simulink model "ModeloCorrea_Cinematico"  (R2023b)
settings: Solver=ode23  StartTime=0.0  StopTime=30  RelTol=1e-3
PreLoadFcn:
  | cargar_datos
model workspace: external: MATLAB File Data\Ensamblaje_Correa_v2_DataFile.m (data not in the file)
undefined symbols (not defined in the file): D, DiscIntNeverNeededParam, Floor, L, R, smiData, X, Y, Z
libraries: sm_lib x464, nesl_utility x23, simulink x8, fl_lib x8, SignalEditorBlockLib x1
(part 2 of 10)

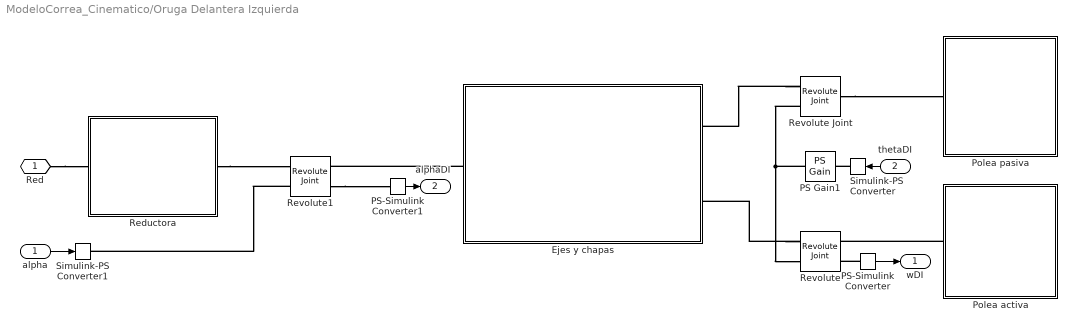
== system ModeloCorrea_Cinematico/Oruga Delantera Izquierda ==
  alpha : Inport
  thetaDI : Inport  Port=2
  Ejes y chapas : Subsystem
      mask Display: image('Ejes y chapas.png');
  PS Gain1 : fl_lib/Physical Signals/Functions/PS Gain  gain=-1
  PS-Simulink Converter : nesl_utility/PS-Simulink Converter  PhysicalDomain=network_engine_domain  SubClassName=ps_output  LeftPortType=input  RightPortType=output  PseudoPeriodic=off  Frequencies=[]  VectorFormat=inherit  Unit=rad/s  AffineConversion=off
  PS-Simulink Converter1 : nesl_utility/PS-Simulink Converter  PhysicalDomain=network_engine_domain  SubClassName=ps_output  LeftPortType=input  RightPortType=output  PseudoPeriodic=off  Frequencies=[]  VectorFormat=inherit  Unit=rad  AffineConversion=off
  Polea activa : Subsystem
      mask Display: image('Polea activa.png');
  Polea pasiva : Subsystem
      mask Display: image('Polea pasiva.png');
  Reductora : Subsystem
      mask Display: image('Reductora.png');
  Revolute : sm_lib/Joints/Revolute Joint  JointMode=Normal  SenseConstraintForce=off  SenseConstraintForceX=off  SenseConstraintForceY=off  SenseConstraintForceZ=off  SenseConstraintTorque=off  SenseConstraintTorqueX=off  SenseConstraintTorqueY=off  SenseConstraintTorqueZ=off  SenseTotalForce=off  SenseTotalForceX=off  SenseTotalForceY=off  SenseTotalForceZ=off  SenseTotalTorque=off  SenseTotalTorqueX=off  SenseTotalTorqueY=off  SenseTotalTorqueZ=off  CompositeWrenchDir=FollowerOnBase  CompositeWrenchFrame=BaseFrame  EquilibriumPosition=0  EquilibriumPositionUnits=deg  SpringStiffness=0  SpringStiffnessUnits=N*m/deg  DampingCoefficient=5e-4  DampingCoefficientUnits=N*m/(deg/s)  TorqueActuationMode=ComputedTorque  MotionActuationMode=InputMotion  SensePosition=off  SenseVelocity=on  SenseAcceleration=off  SenseTorqueForce=off  SenseLowerLimitTorqueForce=off  SenseUpperLimitTorqueForce=off  LowerLimitSpecify=off  LowerLimitBound=-90  LowerLimitBoundUnits=deg  LowerLimitStiffness=1e4  LowerLimitStiffnessUnits=N*m/deg  LowerLimitDamping=10  LowerLimitDampingUnits=N*m/(deg/s)  LowerLimitTransitionRegionWidth=0.1  LowerLimitTransitionRegionWidthUnits=deg  UpperLimitSpecify=off  UpperLimitBound=90  UpperLimitBoundUnits=deg  UpperLimitStiffness=1e4  UpperLimitStiffnessUnits=N*m/deg  UpperLimitDamping=10  UpperLimitDampingUnits=N*m/(deg/s)  UpperLimitTransitionRegionWidth=0.1  UpperLimitTransitionRegionWidthUnits=deg  PositionTargetSpecify=on  PositionTargetPriority=Low  PositionTargetValue=smiData.RevoluteJoint(1).Rz.Pos  PositionTargetValueUnits=deg  VelocityTargetSpecify=off  VelocityTargetPriority=High  VelocityTargetValue=0  VelocityTargetValueUnits=deg/s
  Revolute Joint : sm_lib/Joints/Revolute Joint  JointMode=Normal  SenseConstraintForce=off  SenseConstraintForceX=off  SenseConstraintForceY=off  SenseConstraintForceZ=off  SenseConstraintTorque=off  SenseConstraintTorqueX=off  SenseConstraintTorqueY=off  SenseConstraintTorqueZ=off  SenseTotalForce=off  SenseTotalForceX=off  SenseTotalForceY=off  SenseTotalForceZ=off  SenseTotalTorque=off  SenseTotalTorqueX=off  SenseTotalTorqueY=off  SenseTotalTorqueZ=off  CompositeWrenchDir=FollowerOnBase  CompositeWrenchFrame=BaseFrame  EquilibriumPosition=0  EquilibriumPositionUnits=deg  SpringStiffness=0  SpringStiffnessUnits=N*m/deg  DampingCoefficient=5e-4  DampingCoefficientUnits=N*m/(deg/s)  TorqueActuationMode=ComputedTorque  MotionActuationMode=InputMotion  SensePosition=off  SenseVelocity=off  SenseAcceleration=off  SenseTorqueForce=off  SenseLowerLimitTorqueForce=off  SenseUpperLimitTorqueForce=off  LowerLimitSpecify=off  LowerLimitBound=-90  LowerLimitBoundUnits=deg  LowerLimitStiffness=1e4  LowerLimitStiffnessUnits=N*m/deg  LowerLimitDamping=10  LowerLimitDampingUnits=N*m/(deg/s)  LowerLimitTransitionRegionWidth=0.1  LowerLimitTransitionRegionWidthUnits=deg  UpperLimitSpecify=off  UpperLimitBound=90  UpperLimitBoundUnits=deg  UpperLimitStiffness=1e4  UpperLimitStiffnessUnits=N*m/deg  UpperLimitDamping=10  UpperLimitDampingUnits=N*m/(deg/s)  UpperLimitTransitionRegionWidth=0.1  UpperLimitTransitionRegionWidthUnits=deg  PositionTargetSpecify=off  PositionTargetPriority=High  PositionTargetValue=0  PositionTargetValueUnits=deg  VelocityTargetSpecify=off  VelocityTargetPriority=High  VelocityTargetValue=0  VelocityTargetValueUnits=deg/s
  Revolute1 : sm_lib/Joints/Revolute Joint  JointMode=Normal  SenseConstraintForce=off  SenseConstraintForceX=off  SenseConstraintForceY=off  SenseConstraintForceZ=off  SenseConstraintTorque=off  SenseConstraintTorqueX=off  SenseConstraintTorqueY=off  SenseConstraintTorqueZ=off  SenseTotalForce=off  SenseTotalForceX=off  SenseTotalForceY=off  SenseTotalForceZ=off  SenseTotalTorque=off  SenseTotalTorqueX=off  SenseTotalTorqueY=off  SenseTotalTorqueZ=off  CompositeWrenchDir=FollowerOnBase  CompositeWrenchFrame=BaseFrame  EquilibriumPosition=0  EquilibriumPositionUnits=deg  SpringStiffness=0  SpringStiffnessUnits=N*m/deg  DampingCoefficient=5e-4  DampingCoefficientUnits=N*m/(deg/s)  TorqueActuationMode=ComputedTorque  MotionActuationMode=InputMotion  SensePosition=on  SenseVelocity=off  SenseAcceleration=off  SenseTorqueForce=off  SenseLowerLimitTorqueForce=off  SenseUpperLimitTorqueForce=off  LowerLimitSpecify=on  LowerLimitBound=0  LowerLimitBoundUnits=deg  LowerLimitStiffness=1e4  LowerLimitStiffnessUnits=N*m/deg  LowerLimitDamping=10  LowerLimitDampingUnits=N*m/(deg/s)  LowerLimitTransitionRegionWidth=0.1  LowerLimitTransitionRegionWidthUnits=deg  UpperLimitSpecify=on  UpperLimitBound=90  UpperLimitBoundUnits=deg  UpperLimitStiffness=1e4  UpperLimitStiffnessUnits=N*m/deg  UpperLimitDamping=10  UpperLimitDampingUnits=N*m/(deg/s)  UpperLimitTransitionRegionWidth=0.1  UpperLimitTransitionRegionWidthUnits=deg  PositionTargetSpecify=on  PositionTargetPriority=Low  PositionTargetValue=smiData.RevoluteJoint(2).Rz.Pos  PositionTargetValueUnits=deg  VelocityTargetSpecify=off  VelocityTargetPriority=High  VelocityTargetValue=0  VelocityTargetValueUnits=deg/s
  Simulink-PS Converter : nesl_utility/Simulink-PS Converter  PhysicalDomain=network_engine_domain  SubClassName=ps_input  LeftPortType=input  RightPortType=output  PseudoPeriodic=off  Frequencies=[]  NoiseDistribution=none  NoiseParameters=[]  Unit=1  AffineConversion=off  FilteringAndDerivatives=filter  SimscapeFilterOrder=2  InputFilterTimeConstant=0.001  UdotUserProvided=0
  Simulink-PS Converter1 : nesl_utility/Simulink-PS Converter  PhysicalDomain=network_engine_domain  SubClassName=ps_input  LeftPortType=input  RightPortType=output  PseudoPeriodic=off  Frequencies=[]  NoiseDistribution=none  NoiseParameters=[]  Unit=1  AffineConversion=off  FilteringAndDerivatives=filter  SimscapeFilterOrder=2  InputFilterTimeConstant=0.001  UdotUserProvided=0
  Red : PMIOPort  Side=Left
  wDI : Outport
  alphaDI : Outport  Port=2
  wires:
  thetaDI/1 -> Simulink-PS Converter/1
  PS-Simulink Converter/1 -> wDI/1
  alpha/1 -> Simulink-PS Converter1/1
  PS-Simulink Converter1/1 -> alphaDI/1
  connections:
  Red/RConn1 -- Reductora/LConn1
  Ejes y chapas/LConn1 -- Revolute1/RConn1
  Reductora/RConn1 -- Revolute1/LConn1
  Polea activa/LConn1 -- Revolute/RConn1
  Revolute/LConn1 -- Ejes y chapas/RConn2
  Revolute Joint/RConn1 -- Polea pasiva/LConn1
  Revolute Joint/LConn1 -- Ejes y chapas/RConn1
  PS Gain1/RConn1 -- Revolute/LConn2 -- Revolute Joint/LConn2
  PS-Simulink Converter/LConn1 -- Revolute/RConn2
  Revolute1/LConn2 -- Simulink-PS Converter1/RConn1
  Revolute1/RConn2 -- PS-Simulink Converter1/LConn1
  Simulink-PS Converter/RConn1 -- PS Gain1/LConn1

== system ModeloCorrea_Cinematico/Oruga Trasera Derecha ==
  alpha : Inport
  thetaTD : Inport  Port=2
  Ejes y chapas : Subsystem
      mask Display: image('Ejes y chapas.png');
  PS Gain1 : fl_lib/Physical Signals/Functions/PS Gain  gain=-1
  PS-Simulink Converter : nesl_utility/PS-Simulink Converter  PhysicalDomain=network_engine_domain  SubClassName=ps_output  LeftPortType=input  RightPortType=output  PseudoPeriodic=off  Frequencies=[]  VectorFormat=inherit  Unit=rad/s  AffineConversion=off
  PS-Simulink Converter1 : nesl_utility/PS-Simulink Converter  PhysicalDomain=network_engine_domain  SubClassName=ps_output  LeftPortType=input  RightPortType=output  PseudoPeriodic=off  Frequencies=[]  VectorFormat=inherit  Unit=rad  AffineConversion=off
  Polea activa : Subsystem
      mask Display: image('Polea activa.png');
  Polea pasiva : Subsystem
      mask Display: image('Polea pasiva.png');
  Reductora : Subsystem
      mask Display: image('Reductora.png');
  Revolute : sm_lib/Joints/Revolute Joint  JointMode=Normal  SenseConstraintForce=off  SenseConstraintForceX=off  SenseConstraintForceY=off  SenseConstraintForceZ=off  SenseConstraintTorque=off  SenseConstraintTorqueX=off  SenseConstraintTorqueY=off  SenseConstraintTorqueZ=off  SenseTotalForce=off  SenseTotalForceX=off  SenseTotalForceY=off  SenseTotalForceZ=off  SenseTotalTorque=off  SenseTotalTorqueX=off  SenseTotalTorqueY=off  SenseTotalTorqueZ=off  CompositeWrenchDir=FollowerOnBase  CompositeWrenchFrame=BaseFrame  EquilibriumPosition=0  EquilibriumPositionUnits=deg  SpringStiffness=0  SpringStiffnessUnits=N*m/deg  DampingCoefficient=5e-4  DampingCoefficientUnits=N*m/(deg/s)  TorqueActuationMode=ComputedTorque  MotionActuationMode=InputMotion  SensePosition=off  SenseVelocity=on  SenseAcceleration=off  SenseTorqueForce=off  SenseLowerLimitTorqueForce=off  SenseUpperLimitTorqueForce=off  LowerLimitSpecify=off  LowerLimitBound=-90  LowerLimitBoundUnits=deg  LowerLimitStiffness=1e4  LowerLimitStiffnessUnits=N*m/deg  LowerLimitDamping=10  LowerLimitDampingUnits=N*m/(deg/s)  LowerLimitTransitionRegionWidth=0.1  LowerLimitTransitionRegionWidthUnits=deg  UpperLimitSpecify=off  UpperLimitBound=90  UpperLimitBoundUnits=deg  UpperLimitStiffness=1e4  UpperLimitStiffnessUnits=N*m/deg  UpperLimitDamping=10  UpperLimitDampingUnits=N*m/(deg/s)  UpperLimitTransitionRegionWidth=0.1  UpperLimitTransitionRegionWidthUnits=deg  PositionTargetSpecify=on  PositionTargetPriority=Low  PositionTargetValue=smiData.RevoluteJoint(1).Rz.Pos  PositionTargetValueUnits=deg  VelocityTargetSpecify=off  VelocityTargetPriority=High  VelocityTargetValue=0  VelocityTargetValueUnits=deg/s
  Revolute Joint : sm_lib/Joints/Revolute Joint  JointMode=Normal  SenseConstraintForce=off  SenseConstraintForceX=off  SenseConstraintForceY=off  SenseConstraintForceZ=off  SenseConstraintTorque=off  SenseConstraintTorqueX=off  SenseConstraintTorqueY=off  SenseConstraintTorqueZ=off  SenseTotalForce=off  SenseTotalForceX=off  SenseTotalForceY=off  SenseTotalForceZ=off  SenseTotalTorque=off  SenseTotalTorqueX=off  SenseTotalTorqueY=off  SenseTotalTorqueZ=off  CompositeWrenchDir=FollowerOnBase  CompositeWrenchFrame=BaseFrame  EquilibriumPosition=0  EquilibriumPositionUnits=deg  SpringStiffness=0  SpringStiffnessUnits=N*m/deg  DampingCoefficient=5e-4  DampingCoefficientUnits=N*m/(deg/s)  TorqueActuationMode=ComputedTorque  MotionActuationMode=InputMotion  SensePosition=off  SenseVelocity=off  SenseAcceleration=off  SenseTorqueForce=off  SenseLowerLimitTorqueForce=off  SenseUpperLimitTorqueForce=off  LowerLimitSpecify=off  LowerLimitBound=-90  LowerLimitBoundUnits=deg  LowerLimitStiffness=1e4  LowerLimitStiffnessUnits=N*m/deg  LowerLimitDamping=10  LowerLimitDampingUnits=N*m/(deg/s)  LowerLimitTransitionRegionWidth=0.1  LowerLimitTransitionRegionWidthUnits=deg  UpperLimitSpecify=off  UpperLimitBound=90  UpperLimitBoundUnits=deg  UpperLimitStiffness=1e4  UpperLimitStiffnessUnits=N*m/deg  UpperLimitDamping=10  UpperLimitDampingUnits=N*m/(deg/s)  UpperLimitTransitionRegionWidth=0.1  UpperLimitTransitionRegionWidthUnits=deg  PositionTargetSpecify=off  PositionTargetPriority=High  PositionTargetValue=0  PositionTargetValueUnits=deg  VelocityTargetSpecify=off  VelocityTargetPriority=High  VelocityTargetValue=0  VelocityTargetValueUnits=deg/s
  Revolute1 : sm_lib/Joints/Revolute Joint  JointMode=Normal  SenseConstraintForce=off  SenseConstraintForceX=off  SenseConstraintForceY=off  SenseConstraintForceZ=off  SenseConstraintTorque=off  SenseConstraintTorqueX=off  SenseConstraintTorqueY=off  SenseConstraintTorqueZ=off  SenseTotalForce=off  SenseTotalForceX=off  SenseTotalForceY=off  SenseTotalForceZ=off  SenseTotalTorque=off  SenseTotalTorqueX=off  SenseTotalTorqueY=off  SenseTotalTorqueZ=off  CompositeWrenchDir=FollowerOnBase  CompositeWrenchFrame=BaseFrame  EquilibriumPosition=0  EquilibriumPositionUnits=deg  SpringStiffness=0  SpringStiffnessUnits=N*m/deg  DampingCoefficient=5e-4  DampingCoefficientUnits=N*m/(deg/s)  TorqueActuationMode=ComputedTorque  MotionActuationMode=InputMotion  SensePosition=on  SenseVelocity=off  SenseAcceleration=off  SenseTorqueForce=off  SenseLowerLimitTorqueForce=off  SenseUpperLimitTorqueForce=off  LowerLimitSpecify=on  LowerLimitBound=0  LowerLimitBoundUnits=deg  LowerLimitStiffness=1e4  LowerLimitStiffnessUnits=N*m/deg  LowerLimitDamping=10  LowerLimitDampingUnits=N*m/(deg/s)  LowerLimitTransitionRegionWidth=0.1  LowerLimitTransitionRegionWidthUnits=deg  UpperLimitSpecify=on  UpperLimitBound=90  UpperLimitBoundUnits=deg  UpperLimitStiffness=1e4  UpperLimitStiffnessUnits=N*m/deg  UpperLimitDamping=10  UpperLimitDampingUnits=N*m/(deg/s)  UpperLimitTransitionRegionWidth=0.1  UpperLimitTransitionRegionWidthUnits=deg  PositionTargetSpecify=on  PositionTargetPriority=Low  PositionTargetValue=smiData.RevoluteJoint(2).Rz.Pos  PositionTargetValueUnits=deg  VelocityTargetSpecify=off  VelocityTargetPriority=High  VelocityTargetValue=0  VelocityTargetValueUnits=deg/s
  Simulink-PS Converter : nesl_utility/Simulink-PS Converter  PhysicalDomain=network_engine_domain  SubClassName=ps_input  LeftPortType=input  RightPortType=output  PseudoPeriodic=off  Frequencies=[]  NoiseDistribution=none  NoiseParameters=[]  Unit=1  AffineConversion=off  FilteringAndDerivatives=filter  SimscapeFilterOrder=2  InputFilterTimeConstant=0.001  UdotUserProvided=0
  Simulink-PS Converter1 : nesl_utility/Simulink-PS Converter  PhysicalDomain=network_engine_domain  SubClassName=ps_input  LeftPortType=input  RightPortType=output  PseudoPeriodic=off  Frequencies=[]  NoiseDistribution=none  NoiseParameters=[]  Unit=1  AffineConversion=off  FilteringAndDerivatives=filter  SimscapeFilterOrder=2  InputFilterTimeConstant=0.001  UdotUserProvided=0
  Red : PMIOPort  Side=Left
  wTD : Outport
  alphaTD : Outport  Port=2
  wires:
  thetaTD/1 -> Simulink-PS Converter/1
  PS-Simulink Converter/1 -> wTD/1
  alpha/1 -> Simulink-PS Converter1/1
  PS-Simulink Converter1/1 -> alphaTD/1
  connections:
  Red/RConn1 -- Reductora/LConn1
  Ejes y chapas/LConn1 -- Revolute1/RConn1
  Reductora/RConn1 -- Revolute1/LConn1
  Polea activa/LConn1 -- Revolute/RConn1
  Revolute/LConn1 -- Ejes y chapas/RConn2
  Revolute Joint/RConn1 -- Polea pasiva/LConn1
  Revolute Joint/LConn1 -- Ejes y chapas/RConn1
  Revolute Joint/LConn2 -- Revolute/LConn2 -- PS Gain1/RConn1
  PS-Simulink Converter/LConn1 -- Revolute/RConn2
  Simulink-PS Converter1/RConn1 -- Revolute1/LConn2
  Revolute1/RConn2 -- PS-Simulink Converter1/LConn1
  Simulink-PS Converter/RConn1 -- PS Gain1/LConn1

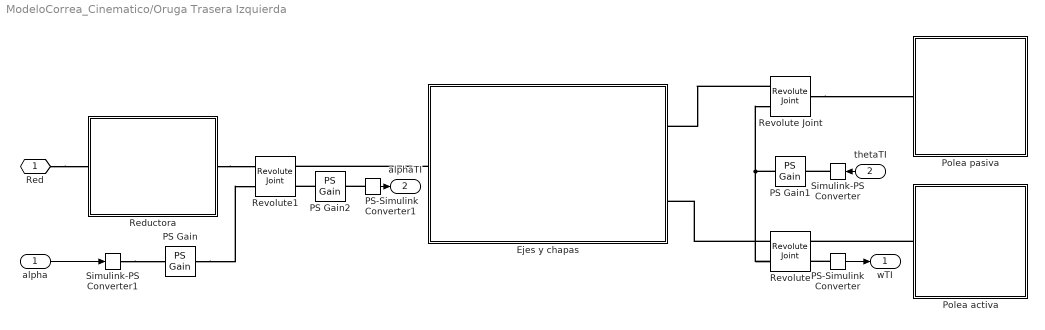
== system ModeloCorrea_Cinematico/Oruga Trasera Izquierda ==
  alpha : Inport
  thetaTI : Inport  Port=2
  Ejes y chapas : Subsystem
      mask Display: image('Ejes y chapas.png');
  PS Gain : fl_lib/Physical Signals/Functions/PS Gain  gain=-1
  PS Gain1 : fl_lib/Physical Signals/Functions/PS Gain  gain=-1
  PS Gain2 : fl_lib/Physical Signals/Functions/PS Gain  gain=-1
  PS-Simulink Converter : nesl_utility/PS-Simulink Converter  PhysicalDomain=network_engine_domain  SubClassName=ps_output  LeftPortType=input  RightPortType=output  PseudoPeriodic=off  Frequencies=[]  VectorFormat=inherit  Unit=rad/s  AffineConversion=off
  PS-Simulink Converter1 : nesl_utility/PS-Simulink Converter  PhysicalDomain=network_engine_domain  SubClassName=ps_output  LeftPortType=input  RightPortType=output  PseudoPeriodic=off  Frequencies=[]  VectorFormat=inherit  Unit=rad  AffineConversion=off
  Polea activa : Subsystem
      mask Display: image('Polea activa.png');
  Polea pasiva : Subsystem
      mask Display: image('Polea pasiva.png');
  Reductora : Subsystem
      mask Display: image('Reductora.png');
  Revolute : sm_lib/Joints/Revolute Joint  JointMode=Normal  SenseConstraintForce=off  SenseConstraintForceX=off  SenseConstraintForceY=off  SenseConstraintForceZ=off  SenseConstraintTorque=off  SenseConstraintTorqueX=off  SenseConstraintTorqueY=off  SenseConstraintTorqueZ=off  SenseTotalForce=off  SenseTotalForceX=off  SenseTotalForceY=off  SenseTotalForceZ=off  SenseTotalTorque=off  SenseTotalTorqueX=off  SenseTotalTorqueY=off  SenseTotalTorqueZ=off  CompositeWrenchDir=FollowerOnBase  CompositeWrenchFrame=BaseFrame  EquilibriumPosition=0  EquilibriumPositionUnits=deg  SpringStiffness=0  SpringStiffnessUnits=N*m/deg  DampingCoefficient=5e-4  DampingCoefficientUnits=N*m/(deg/s)  TorqueActuationMode=ComputedTorque  MotionActuationMode=InputMotion  SensePosition=off  SenseVelocity=on  SenseAcceleration=off  SenseTorqueForce=off  SenseLowerLimitTorqueForce=off  SenseUpperLimitTorqueForce=off  LowerLimitSpecify=off  LowerLimitBound=-90  LowerLimitBoundUnits=deg  LowerLimitStiffness=1e4  LowerLimitStiffnessUnits=N*m/deg  LowerLimitDamping=10  LowerLimitDampingUnits=N*m/(deg/s)  LowerLimitTransitionRegionWidth=0.1  LowerLimitTransitionRegionWidthUnits=deg  UpperLimitSpecify=off  UpperLimitBound=90  UpperLimitBoundUnits=deg  UpperLimitStiffness=1e4  UpperLimitStiffnessUnits=N*m/deg  UpperLimitDamping=10  UpperLimitDampingUnits=N*m/(deg/s)  UpperLimitTransitionRegionWidth=0.1  UpperLimitTransitionRegionWidthUnits=deg  PositionTargetSpecify=on  PositionTargetPriority=Low  PositionTargetValue=smiData.RevoluteJoint(1).Rz.Pos  PositionTargetValueUnits=deg  VelocityTargetSpecify=off  VelocityTargetPriority=High  VelocityTargetValue=0  VelocityTargetValueUnits=deg/s
  Revolute Joint : sm_lib/Joints/Revolute Joint  JointMode=Normal  SenseConstraintForce=off  SenseConstraintForceX=off  SenseConstraintForceY=off  SenseConstraintForceZ=off  SenseConstraintTorque=off  SenseConstraintTorqueX=off  SenseConstraintTorqueY=off  SenseConstraintTorqueZ=off  SenseTotalForce=off  SenseTotalForceX=off  SenseTotalForceY=off  SenseTotalForceZ=off  SenseTotalTorque=off  SenseTotalTorqueX=off  SenseTotalTorqueY=off  SenseTotalTorqueZ=off  CompositeWrenchDir=FollowerOnBase  CompositeWrenchFrame=BaseFrame  EquilibriumPosition=0  EquilibriumPositionUnits=deg  SpringStiffness=0  SpringStiffnessUnits=N*m/deg  DampingCoefficient=5e-4  DampingCoefficientUnits=N*m/(deg/s)  TorqueActuationMode=ComputedTorque  MotionActuationMode=InputMotion  SensePosition=off  SenseVelocity=off  SenseAcceleration=off  SenseTorqueForce=off  SenseLowerLimitTorqueForce=off  SenseUpperLimitTorqueForce=off  LowerLimitSpecify=off  LowerLimitBound=-90  LowerLimitBoundUnits=deg  LowerLimitStiffness=1e4  LowerLimitStiffnessUnits=N*m/deg  LowerLimitDamping=10  LowerLimitDampingUnits=N*m/(deg/s)  LowerLimitTransitionRegionWidth=0.1  LowerLimitTransitionRegionWidthUnits=deg  UpperLimitSpecify=off  UpperLimitBound=90  UpperLimitBoundUnits=deg  UpperLimitStiffness=1e4  UpperLimitStiffnessUnits=N*m/deg  UpperLimitDamping=10  UpperLimitDampingUnits=N*m/(deg/s)  UpperLimitTransitionRegionWidth=0.1  UpperLimitTransitionRegionWidthUnits=deg  PositionTargetSpecify=off  PositionTargetPriority=High  PositionTargetValue=0  PositionTargetValueUnits=deg  VelocityTargetSpecify=off  VelocityTargetPriority=High  VelocityTargetValue=0  VelocityTargetValueUnits=deg/s
  Revolute1 : sm_lib/Joints/Revolute Joint  JointMode=Normal  SenseConstraintForce=off  SenseConstraintForceX=off  SenseConstraintForceY=off  SenseConstraintForceZ=off  SenseConstraintTorque=off  SenseConstraintTorqueX=off  SenseConstraintTorqueY=off  SenseConstraintTorqueZ=off  SenseTotalForce=off  SenseTotalForceX=off  SenseTotalForceY=off  SenseTotalForceZ=off  SenseTotalTorque=off  SenseTotalTorqueX=off  SenseTotalTorqueY=off  SenseTotalTorqueZ=off  CompositeWrenchDir=FollowerOnBase  CompositeWrenchFrame=BaseFrame  EquilibriumPosition=0  EquilibriumPositionUnits=deg  SpringStiffness=0  SpringStiffnessUnits=N*m/deg  DampingCoefficient=5e-4  DampingCoefficientUnits=N*m/(deg/s)  TorqueActuationMode=ComputedTorque  MotionActuationMode=InputMotion  SensePosition=on  SenseVelocity=off  SenseAcceleration=off  SenseTorqueForce=off  SenseLowerLimitTorqueForce=off  SenseUpperLimitTorqueForce=off  LowerLimitSpecify=on  LowerLimitBound=0  LowerLimitBoundUnits=deg  LowerLimitStiffness=1e4  LowerLimitStiffnessUnits=N*m/deg  LowerLimitDamping=10  LowerLimitDampingUnits=N*m/(deg/s)  LowerLimitTransitionRegionWidth=0.1  LowerLimitTransitionRegionWidthUnits=deg  UpperLimitSpecify=on  UpperLimitBound=90  UpperLimitBoundUnits=deg  UpperLimitStiffness=1e4  UpperLimitStiffnessUnits=N*m/deg  UpperLimitDamping=10  UpperLimitDampingUnits=N*m/(deg/s)  UpperLimitTransitionRegionWidth=0.1  UpperLimitTransitionRegionWidthUnits=deg  PositionTargetSpecify=on  PositionTargetPriority=Low  PositionTargetValue=smiData.RevoluteJoint(2).Rz.Pos  PositionTargetValueUnits=deg  VelocityTargetSpecify=off  VelocityTargetPriority=High  VelocityTargetValue=0  VelocityTargetValueUnits=deg/s
  Simulink-PS Converter : nesl_utility/Simulink-PS Converter  PhysicalDomain=network_engine_domain  SubClassName=ps_input  LeftPortType=input  RightPortType=output  PseudoPeriodic=off  Frequencies=[]  NoiseDistribution=none  NoiseParameters=[]  Unit=1  AffineConversion=off  FilteringAndDerivatives=filter  SimscapeFilterOrder=2  InputFilterTimeConstant=0.001  UdotUserProvided=0
  Simulink-PS Converter1 : nesl_utility/Simulink-PS Converter  PhysicalDomain=network_engine_domain  SubClassName=ps_input  LeftPortType=input  RightPortType=output  PseudoPeriodic=off  Frequencies=[]  NoiseDistribution=none  NoiseParameters=[]  Unit=1  AffineConversion=off  FilteringAndDerivatives=filter  SimscapeFilterOrder=2  InputFilterTimeConstant=0.001  UdotUserProvided=0
  Red : PMIOPort  Side=Left
  wTI : Outport
  alphaTI : Outport  Port=2
  wires:
  thetaTI/1 -> Simulink-PS Converter/1
  PS-Simulink Converter/1 -> wTI/1
  alpha/1 -> Simulink-PS Converter1/1
  PS-Simulink Converter1/1 -> alphaTI/1
  connections:
  Red/RConn1 -- Reductora/LConn1
  Ejes y chapas/LConn1 -- Revolute1/RConn1
  Reductora/RConn1 -- Revolute1/LConn1
  Polea activa/LConn1 -- Revolute/RConn1
  Revolute/LConn1 -- Ejes y chapas/RConn2
  Revolute Joint/RConn1 -- Polea pasiva/LConn1
  PS Gain/RConn1 -- Revolute1/LConn2
  Revolute Joint/LConn1 -- Ejes y chapas/RConn1
  Revolute/LConn2 -- Revolute Joint/LConn2 -- PS Gain1/RConn1
  PS-Simulink Converter/LConn1 -- Revolute/RConn2
  PS-Simulink Converter1/LConn1 -- PS Gain2/RConn1
  Simulink-PS Converter1/RConn1 -- PS Gain/LConn1
  Simulink-PS Converter/RConn1 -- PS Gain1/LConn1
  PS Gain2/LConn1 -- Revolute1/RConn2

== system ModeloCorrea_Cinematico/Suelo ==
  Brick Solid : sm_lib/Body Elements/Brick Solid  GraphicAmbientColor=[0.15 0.15 0.15 1.0]  BasedOnType=Density  BrickDimensions=[Floor.l , Floor.w , Floor.h]  BrickDimensionsUnits=m  CenterOfMass=[0 0 0]  CenterOfMassUnits=m  GraphicDiffuseColor=[0.8 0.8 0.8]  Density=1000  DensityUnits=kg/m^3  DoExposeReferenceFrame=on  GraphicEmissiveColor=[0.0 0.0 0.0 1.0]  ExportEntireGeometry=off  SerializedFrames=<Frames/>  MarkerShape=Sphere  MarkerSize=10  GraphicType=FromGeometry  InertiaType=CalculateFromGeometry  Mass=1  MassUnits=kg  MomentsOfInertia=[1 1 1]  MomentsOfInertiaUnits=kg*m^2  GraphicOpacity=1.0  ProductsOfInertia=[0 0 0]  ProductsOfInertiaUnits=kg*m^2  GraphicShininess=75  GraphicSpecularColor=[0.5 0.5 0.5 1.0]  GraphicVisPropType=SimpleVisualProperties
  Extruded Solid : sm_lib/Body Elements/Extruded Solid  GraphicAmbientColor=[0.15 0.15 0.15 1.0]  BasedOnType=Density  CenterOfMass=[0 0 0]  CenterOfMassUnits=m  GraphicDiffuseColor=[0.4 0.4 0.4]  ExportConvexHullGeometry=off  ExtrusionCrossSection=Grid.extr_data  ExtrusionCrossSectionUnits=m  Density=1000  DensityUnits=kg/m^3  DoExposeReferenceFrame=on  GraphicEmissiveColor=[0.0 0.0 0.0 1.0]  ExportEntireGeometry=off  ExtrusionLength=Floor.h*1.005  ExtrusionLengthUnits=m  ExtrusionType=General  SerializedFrames=<Frames/>  MarkerShape=Sphere  MarkerSize=10  GraphicType=FromGeometry  InertiaType=CalculateFromGeometry  Mass=1  MassUnits=kg  MomentsOfInertia=[1 1 1]  MomentsOfInertiaUnits=kg*m^2  PolygonNumSides=3  GraphicOpacity=1.0  PolygonOuterRadius=1  PolygonOuterRadiusUnits=m  ProductsOfInertia=[0 0 0]  ProductsOfInertiaUnits=kg*m^2  GraphicShininess=75  GraphicSpecularColor=[0.5 0.5 0.5 1.0]  GraphicVisPropType=SimpleVisualProperties
  Extruded Solid1 : sm_lib/Body Elements/Extruded Solid  GraphicAmbientColor=[0.15 0.15 0.15 1.0]  BasedOnType=Density  CenterOfMass=[0 0 0]  CenterOfMassUnits=m  GraphicDiffuseColor=[0.4 0.4 0.4]  ExportConvexHullGeometry=off  ExtrusionCrossSection=Grid.extr_data  ExtrusionCrossSectionUnits=m  Density=1000  DensityUnits=kg/m^3  DoExposeReferenceFrame=on  GraphicEmissiveColor=[0.0 0.0 0.0 1.0]  ExportEntireGeometry=off  ExtrusionLength=Floor.h*1.005  ExtrusionLengthUnits=m  ExtrusionType=General  SerializedFrames=<Frames/>  MarkerShape=Sphere  MarkerSize=10  GraphicType=FromGeometry  InertiaType=CalculateFromGeometry  Mass=1  MassUnits=kg  MomentsOfInertia=[1 1 1]  MomentsOfInertiaUnits=kg*m^2  PolygonNumSides=3  GraphicOpacity=1.0  PolygonOuterRadius=1  PolygonOuterRadiusUnits=m  ProductsOfInertia=[0 0 0]  ProductsOfInertiaUnits=kg*m^2  GraphicShininess=75  GraphicSpecularColor=[0.5 0.5 0.5 1.0]  GraphicVisPropType=SimpleVisualProperties
  Rigid Transform1 : sm_lib/Frames and Transforms/Rigid Transform  TranslationMethod=None  TranslationStandardOffset=0  TranslationStandardOffsetUnits=m  TranslationStandardAxis=+Z  TranslationCartesianOffset=[0 0 0]  TranslationCartesianOffsetUnits=m  TranslationROffset=0  TranslationROffsetUnits=m  TranslationZOffset=0  TranslationZOffsetUnits=m  TranslationThetaOffset=0  TranslationThetaOffsetUnits=deg  RotationMethod=StandardAxis  RotationAngleUnits=deg  RotationStandardAxis=+Z  RotationAngle=90  RotationArbitraryAxis=[0 0 1]  FollAlignAxisA=+X  BaseAlignAxisA=+Y  FollAlignAxisB=+Y  BaseAlignAxisB=+Z  RotationSequenceAxes=FollowerAxes  RotationSequence=XYX  RotationSequenceAngles=[90 90 0]  RotationSequenceAnglesUnits=deg  RotationMatrix=[1 0 0; 0 1 0; 0 0 1]  Quaternion=[1 0 0 0]
  Input : PMIOPort  Side=Left
  connections:
  Extruded Solid/RConn1 -- Rigid Transform1/LConn1
  Input/RConn1 -- Brick Solid/RConn1 -- Extruded Solid1/RConn1 -- Rigid Transform1/RConn1

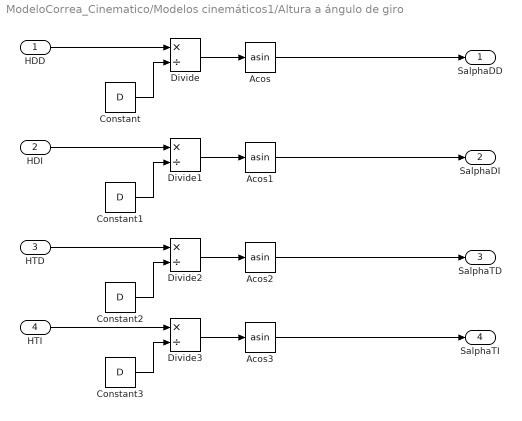
== system ModeloCorrea_Cinematico/Modelos cinemáticos1/Altura a ángulo de giro ==
  HDD : Inport
  HDI : Inport  Port=2
  HTD : Inport  Port=3
  HTI : Inport  Port=4
  Acos{,1..3} (4 alike) : Trigonometry  Operator=asin
  Constant{,1..3} (4 alike) : Constant  Value=D
  Divide{,1..3} (4 alike) : Product  Inputs=*/  RndMeth=Zero  SaturateOnIntegerOverflow=on
  SalphaDD : Outport
  SalphaDI : Outport  Port=2
  SalphaTD : Outport  Port=3
  SalphaTI : Outport  Port=4
  wires:
  Constant/1 -> Divide/2
  Divide/1 -> Acos/1
  Acos/1 -> SalphaDD/1
  HDD/1 -> Divide/1
  Divide1/1 -> Acos1/1
  Constant1/1 -> Divide1/2
  HDI/1 -> Divide1/1
  Acos1/1 -> SalphaDI/1
  Divide2/1 -> Acos2/1
  Constant2/1 -> Divide2/2
  HTD/1 -> Divide2/1
  Acos2/1 -> SalphaTD/1
  Divide3/1 -> Acos3/1
  Constant3/1 -> Divide3/2
  HTI/1 -> Divide3/1
  Acos3/1 -> SalphaTI/1

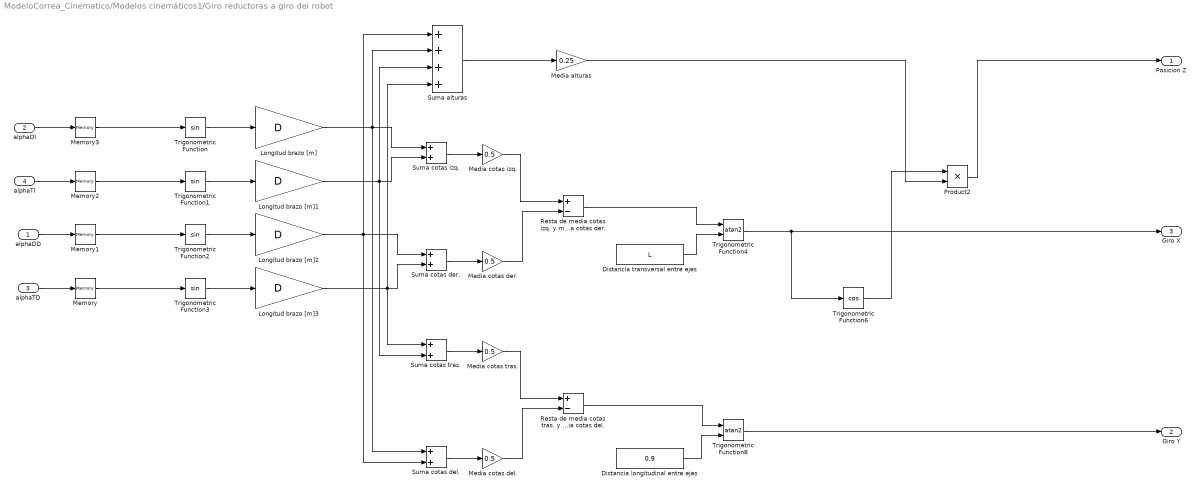
== system ModeloCorrea_Cinematico/Modelos cinemáticos1/Giro reductoras a giro del robot ==
  alphaDD : Inport
  alphaDI : Inport  Port=2
  alphaTD : Inport  Port=3
  alphaTI : Inport  Port=4
  Distancia longitudinal entre ejes : Constant  Value=0.9
  Distancia transversal entre ejes : Constant  Value=L
  Longitud brazo [m]{,1..3} (4 alike) : Gain  Gain=D
  Media alturas : Gain  Gain=0.25
  Media cotas del. : Gain  Gain=0.5
  Media cotas der. : Gain  Gain=0.5
  Media cotas izq. : Gain  Gain=0.5
  Media cotas tras. : Gain  Gain=0.5
  Memory{,1..3} (4 alike) : Memory
  Product2 : Product  Inputs=**
  Resta de media cotas izq. y media cotas der. : Sum  Inputs=+-
  Resta de media cotas tras. y media cotas del. : Sum  Inputs=+-
  Suma alturas : Sum  Inputs=++++
  Suma cotas del. : Sum
  Suma cotas der. : Sum
  Suma cotas izq. : Sum
  Suma cotas tras. : Sum
  Trigonometric Function{,1..3} (4 alike) : Trigonometry
  Trigonometric Function4 : Trigonometry  Operator=atan2
  Trigonometric Function6 : Trigonometry  Operator=cos
  Trigonometric Function8 : Trigonometry  Operator=atan2
  Posicion Z : Outport
  Giro Y : Outport  Port=2
  Giro X : Outport  Port=3
  wires:
  Trigonometric Function/1 -> Longitud brazo [m]/1
  Trigonometric Function1/1 -> Longitud brazo [m]1/1
  Trigonometric Function2/1 -> Longitud brazo [m]2/1
  Trigonometric Function3/1 -> Longitud brazo [m]3/1
  Longitud brazo [m]/1 -> Suma alturas/2, Suma cotas del./1, Suma cotas izq./1
  Longitud brazo [m]3/1 -> Suma alturas/4, Suma cotas tras./1, Suma cotas der./2
  Suma cotas der./1 -> Media cotas der./1
  Suma cotas izq./1 -> Media cotas izq./1
  Media cotas der./1 -> Resta de media cotas izq. y media cotas der./2
  Media cotas izq./1 -> Resta de media cotas izq. y media cotas der./1
  Resta de media cotas izq. y media cotas der./1 -> Trigonometric Function4/1
  Suma cotas del./1 -> Media cotas del./1
  Suma cotas tras./1 -> Media cotas tras./1
  Media cotas del./1 -> Resta de media cotas tras. y media cotas del./2
  Media cotas tras./1 -> Resta de media cotas tras. y media cotas del./1
  Longitud brazo [m]1/1 -> Suma alturas/3, Suma cotas tras./2, Suma cotas izq./2
  Distancia transversal entre ejes/1 -> Trigonometric Function4/2
  Resta de media cotas tras. y media cotas del./1 -> Trigonometric Function8/1
  Distancia longitudinal entre ejes/1 -> Trigonometric Function8/2
  Suma alturas/1 -> Media alturas/1
  Media alturas/1 -> Product2/2
  Trigonometric Function6/1 -> Product2/1
  Longitud brazo [m]2/1 -> Suma alturas/1, Suma cotas del./2, Suma cotas der./1
  Memory/1 -> Trigonometric Function3/1
  Memory1/1 -> Trigonometric Function2/1
  Memory2/1 -> Trigonometric Function1/1
  Memory3/1 -> Trigonometric Function/1
  alphaDI/1 -> Memory3/1
  alphaTI/1 -> Memory2/1
  alphaTD/1 -> Memory/1
  alphaDD/1 -> Memory1/1
  Trigonometric Function8/1 -> Giro Y/1
  Trigonometric Function4/1 -> Giro X/1, Trigonometric Function6/1
  Product2/1 -> Posicion Z/1

== system ModeloCorrea_Cinematico/Modelos cinemáticos1/Modelo Cinematico Inverso ==
  "[v,w]" : Inport
  Gain : Gain  Gain=[1 -L/2; 1 L/2]  Multiplication=Matrix(K*u) (u vector)
  "[vi;vd] m/s" : Outport  VectorParamsAs1DForOutWhenUnconnected=off
  wires:
  "[v,w]"/1 -> Gain/1
  Gain/1 -> "[vi;vd] m/s"/1

== system ModeloCorrea_Cinematico/Modelos cinemáticos1/Modelo Cinemático Directo ==
  wDD : Inport
  wDI : Inport  Port=2
  wTD : Inport  Port=3
  wTI : Inport  Port=4
  Constant : Constant  Value=2
  Divide : Product  Inputs=*/
  Divide1 : Product  Inputs=*/
  Gain : Gain  Gain=R
  Gain1 : Gain  Gain=[1/2 1/2; -1/L 1/L]  Multiplication=Matrix(K*u) (u vector)
  Gain2 : Gain  Gain=R
  Mux : Mux  Inputs=2
  Sum : Sum  Inputs=|++
  Sum1 : Sum  Inputs=|++
  "[v,w]" : Outport  VectorParamsAs1DForOutWhenUnconnected=off
  wires:
  Mux/1 -> Gain1/1
  Gain1/1 -> "[v,w]"/1
  Divide1/1 -> Gain2/1
  Divide/1 -> Gain/1
  wTI/1 -> Sum/2
  wDI/1 -> Sum/1
  wDD/1 -> Sum1/1
  Constant/1 -> Divide/2, Divide1/2
  Sum/1 -> Divide1/1
  Sum1/1 -> Divide/1
  wTD/1 -> Sum1/2
  Gain/1 -> Mux/1
  Gain2/1 -> Mux/2

== system ModeloCorrea_Cinematico/Modelos cinemáticos1/Odometría ==
  "[v,w]" : Inport
  Cos : Trigonometry  Operator=cos
  Demux : Demux  Outputs=2
  Demux1 : Demux  Outputs=3
  Discrete-Time Integrator : DiscreteIntegrator  SampleTime=-1  ICPrevOutput=DiscIntNeverNeededParam  ICPrevScaledInput=DiscIntNeverNeededParam
  Multiply : Product
  Multiply1 : Product
  Mux : Mux  Inputs=3
  Sin : Trigonometry
  x : Outport
  y : Outport  Port=2
  theta : Outport  Port=3
  wires:
  "[v,w]"/1 -> Demux/1
  Demux/1 -> Multiply/2, Multiply1/1
  Sin/1 -> Multiply1/2
  Cos/1 -> Multiply/1
  Multiply/1 -> Mux/1
  Multiply1/1 -> Mux/2
  Demux/2 -> Mux/3
  Mux/1 -> Discrete-Time Integrator/1
  Demux1/3 -> Sin/1, Cos/1, theta/1
  Discrete-Time Integrator/1 -> Demux1/1
  Demux1/2 -> y/1
  Demux1/1 -> x/1

== system ModeloCorrea_Cinematico/Modelos cinemáticos1/Velocidad a ángulo ==
  "[vi,vd]" : Inport
  Demux : Demux  Outputs=2
  Gain : Gain  Gain=1/R
  Gain1 : Gain  Gain=1/R
  Integrator : Integrator
  Integrator1 : Integrator
  ThetaDI : Outport
  ThetaTI : Outport  Port=2
  ThetaDD : Outport  Port=3
  ThetaTD : Outport  Port=4
  wires:
  "[vi,vd]"/1 -> Demux/1
  Demux/1 -> Gain/1
  Demux/2 -> Gain1/1
  Gain/1 -> Integrator/1
  Gain1/1 -> Integrator1/1
  Integrator/1 -> ThetaTI/1, ThetaDI/1
  Integrator1/1 -> ThetaTD/1, ThetaDD/1

== system ModeloCorrea_Cinematico/Modulador/Subsystem ==
  In1 : Inport
  In2 : Inport  Port=2
  Add : Sum
  Constant4 : Constant  Value=0.02635
  Constant5 : Constant  Value=0.3
  Memory1 : Memory  InitialCondition=0.02635
  Rate Limiter : RateLimiter  RisingSlewLimit=0.1  FallingSlewLimit=-0.1  SampleTimeMode=inherited  InitialCondition=0.02635
  Switch1 : Switch  Criteria=u2 > Threshold  Threshold=1  SaturateOnIntegerOverflow=off  InputSameDT=off
  Switch2 : Switch  Criteria=u2 ~= 0  SaturateOnIntegerOverflow=off  InputSameDT=off
  Output : Outport
  wires:
  In1/1 -> Add/1
  In2/1 -> Add/2
  Constant4/1 -> Switch1/1
  Constant5/1 -> Switch1/3
  Switch2/1 -> Rate Limiter/1
  Memory1/1 -> Switch2/3
  Add/1 -> Switch2/2, Switch1/2
  Switch1/1 -> Switch2/1
  Rate Limiter/1 -> Memory1/1, Output/1

== system ModeloCorrea_Cinematico/Modulador/Subsystem1 ==
  In1 : Inport
  In2 : Inport  Port=2
  Add : Sum
  Constant4 : Constant  Value=0.02635
  Constant5 : Constant  Value=0.3
  Memory1 : Memory  InitialCondition=0.02635
  Rate Limiter : RateLimiter  RisingSlewLimit=0.1  FallingSlewLimit=-0.1  SampleTimeMode=inherited  InitialCondition=0.02635
  Switch1 : Switch  Criteria=u2 > Threshold  Threshold=1  SaturateOnIntegerOverflow=off  InputSameDT=off
  Switch2 : Switch  Criteria=u2 ~= 0  SaturateOnIntegerOverflow=off  InputSameDT=off
  Output : Outport
  wires:
  In1/1 -> Add/1
  In2/1 -> Add/2
  Constant4/1 -> Switch1/1
  Constant5/1 -> Switch1/3
  Add/1 -> Switch2/2, Switch1/2
  Switch1/1 -> Switch2/1
  Rate Limiter/1 -> Memory1/1, Output/1
  Switch2/1 -> Rate Limiter/1
  Memory1/1 -> Switch2/3

== system ModeloCorrea_Cinematico/Modulador/Subsystem2 ==
  In1 : Inport
  In2 : Inport  Port=2
  Add : Sum
  Constant4 : Constant  Value=0.02635
  Constant5 : Constant  Value=0.3
  Memory1 : Memory  InitialCondition=0.02635
  Rate Limiter : RateLimiter  RisingSlewLimit=0.1  FallingSlewLimit=-0.1  SampleTimeMode=inherited  InitialCondition=0.02635
  Switch1 : Switch  Criteria=u2 > Threshold  Threshold=1  SaturateOnIntegerOverflow=off  InputSameDT=off
  Switch2 : Switch  Criteria=u2 ~= 0  SaturateOnIntegerOverflow=off  InputSameDT=off
  Output : Outport
  wires:
  In1/1 -> Add/1
  In2/1 -> Add/2
  Constant4/1 -> Switch1/1
  Constant5/1 -> Switch1/3
  Add/1 -> Switch2/2, Switch1/2
  Switch1/1 -> Switch2/1
  Rate Limiter/1 -> Memory1/1, Output/1
  Switch2/1 -> Rate Limiter/1
  Memory1/1 -> Switch2/3

== system ModeloCorrea_Cinematico/Modulador/Subsystem3 ==
  In1 : Inport
  In2 : Inport  Port=2
  Add : Sum
  Constant4 : Constant  Value=0.02635
  Constant5 : Constant  Value=0.3
  Memory2 : Memory  InitialCondition=0.02635
  Rate Limiter : RateLimiter  RisingSlewLimit=0.1  FallingSlewLimit=-0.1  SampleTimeMode=inherited  InitialCondition=0.02635
  Switch1 : Switch  Criteria=u2 > Threshold  Threshold=1  SaturateOnIntegerOverflow=off  InputSameDT=off
  Switch2 : Switch  Criteria=u2 ~= 0  SaturateOnIntegerOverflow=off  InputSameDT=off
  Output1 : Outport
  wires:
  In1/1 -> Add/1
  In2/1 -> Add/2
  Constant4/1 -> Switch1/1
  Constant5/1 -> Switch1/3
  Add/1 -> Switch2/2, Switch1/2
  Switch1/1 -> Switch2/1
  Rate Limiter/1 -> Memory2/1, Output1/1
  Switch2/1 -> Rate Limiter/1
  Memory2/1 -> Switch2/3
